simulink model "sector_selection"  (R2015a)
settings: Solver=ode3  StartTime=0.0  StopTime=0.5  FixedStep=Ts  RelTol=1e-3
settings Model: Creator=rblan  LastModifiedBy=rblan

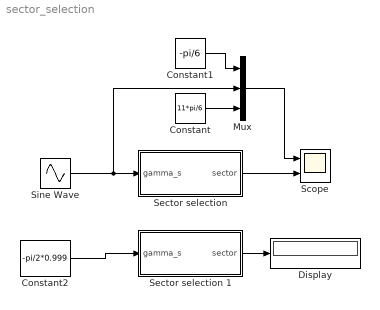
== system sector_selection ==
  Constant : Constant  Value=11*pi/6
  Constant1 : Constant  Value=-pi/6
  Constant2 : Constant  Value=-pi/2*0.999
  Display : Display
  Mux : Mux  Inputs=3
  Scope : Scope  NumInputPorts=2
      settings: YMin=-2~0  YMax=5~12
  "Sector selection " : Subsystem
  Sector selection 1 : Subsystem
  Sine Wave : Sin  Amplitude=pi*0.999  Bias=5*pi/6  Frequency=2*pi*50  SampleTime=0
  wires:
  "Sector selection "/1("sector ") -> Scope/2
  Sine Wave/1 -> "Sector selection "/1(gamma_s), Mux/2
  Mux/1 -> Scope/1
  Constant/1 -> Mux/3
  Constant1/1 -> Mux/1
  Constant2/1 -> Sector selection 1/1(gamma_s)
  Sector selection 1/1("sector ") -> Display/1

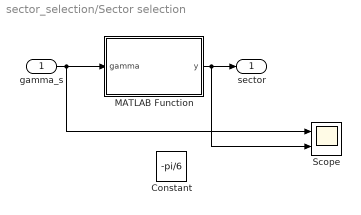
== system sector_selection/Sector selection  ==
  gamma_s : Inport
  Constant : Constant  Value=-pi/6
  MATLAB Function : MATLAB Function  TreatAsAtomicUnit=on
  Scope : Scope  NumInputPorts=2
      settings: ShowLegends=on  YMin=-2~10  YMax=5~12  SaveName=ScopeData10
  "sector " : Outport
  wires:
  MATLAB Function/1(y) -> Scope/2, "sector "/1
  gamma_s/1 -> Scope/1, MATLAB Function/1(gamma)

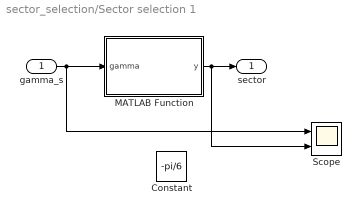
== system sector_selection/Sector selection 1 ==
  gamma_s : Inport
  Constant : Constant  Value=-pi/6
  MATLAB Function : MATLAB Function  TreatAsAtomicUnit=on
  Scope : Scope  NumInputPorts=2
      settings: ShowLegends=on  YMin=-2~10  YMax=5~12  SaveName=ScopeData10
  "sector " : Outport
  wires:
  MATLAB Function/1(y) -> Scope/2, "sector "/1
  gamma_s/1 -> Scope/1, MATLAB Function/1(gamma)

== matlab function sector_selection/Sector selection 1/MATLAB Function ==
  data: gamma input; y output
function y = fcn(gamma)
%#codegen

% persistent n ; 
% n = 1 ; 
% 
% % gamma
% up = (n-1)*pi/6  ; 
% down = (n-2)*pi/6 ;  
% % n 
% 
% 
% if (n>=11 && gamma <0 ) 
%     gamma = gamma + 2*pi ; 
% end 
% while (down >=gamma || gamma > up) 
%     if n==12 
%         n=1 ; 
%     else 
%         n=n+1  
%     end
%    if (n>=11 && gamma <0 ) 
%     gamma = gamma + 2*pi ; 
%    end 
%     up = (n-1)*pi/6  
%     down = (n-2)*pi/6 
%     gamma
% end 
% y=n 


% gamma
if (gamma < -pi/6) 
    gamma = gamma +2*pi ; 
end 
n= 1 ; 
up = (n-1)*pi/6  ; 
down = (n-2)*pi/6 ;  
 
while (down >=gamma || gamma > up) 
    if n==12 
        n=1 ; 
    else 
        n=n+1 ; 
    end
    up = (n-1)*pi/6  ;
    down = (n-2)*pi/6 ;
end 
y=n ;

== matlab function sector_selection/Sector selection /MATLAB Function ==
  data: gamma input; y output
function y = fcn(gamma)
%#codegen

% persistent n ; 
% n = 1 ; 
% 
% % gamma
% up = (n-1)*pi/6  ; 
% down = (n-2)*pi/6 ;  
% % n 
% 
% 
% if (n>=11 && gamma <0 ) 
%     gamma = gamma + 2*pi ; 
% end 
% while (down >=gamma || gamma > up) 
%     if n==12 
%         n=1 ; 
%     else 
%         n=n+1  
%     end
%    if (n>=11 && gamma <0 ) 
%     gamma = gamma + 2*pi ; 
%    end 
%     up = (n-1)*pi/6  
%     down = (n-2)*pi/6 
%     gamma
% end 
% y=n 


% gamma
if (gamma < -pi/6) 
    gamma = gamma +2*pi ; 
end 

n= 1 ; 
up = (n-1)*pi/6  ; 
down = (n-2)*pi/6 ;  
 
while (down >=gamma || gamma > up) 
    if n==12 
        n=1 ; 
    else 
        n=n+1 ; 
    end
    up = (n-1)*pi/6  ;
    down = (n-2)*pi/6 ;
end 
y=n ;
